simulink model "Utkarsh_2005574_R_W1_P1"  (R2021a)
settings: Solver=VariableStepAuto  StartTime=0.0  StopTime=10.0  RelTol=1e-3
PostLoadFcn:
  | M1=100;
  | K1=50;
  | b=50;
  | M2=40;
  | K12=10;
settings Model: Creator=Utkarsh Anand  LastModifiedBy=Utkarsh Anand

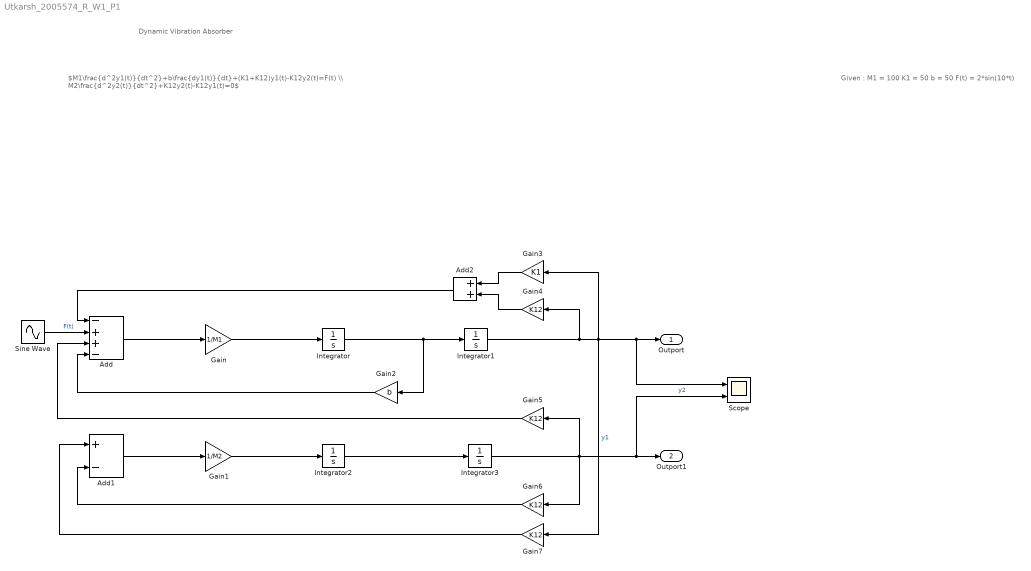
== system Utkarsh_2005574_R_W1_P1 ==
  note: Given :
      | M1 = 100
      | K1 = 50
      | b = 50
      | F(t) = 2*sin(10*t)
  note: $M1\frac{d^2y1(t)}{dt^2}+b\frac{dy1(t)}{dt}+(K1+K12)y1(t)-K12y2(t)=F(t) \\ M2\frac{d^2y2(t)}{dt^2}+K12y2(t)-K12y1(t)=0$
  note: Dynamic Vibration Absorber
  Add : Sum  Inputs=-++-
  Add1 : Sum  Inputs=+-
  Add2 : Sum
  Gain : Gain  Gain=1/M1
  Gain1 : Gain  Gain=1/M2
  Gain2 : Gain  Gain=b
  Gain3 : Gain  Gain=K1
  Gain{4..7} (4 alike) : Gain  Gain=K12
  Integrator{,1..3} (4 alike) : Integrator
  Scope : Scope  NumInputPorts=2
  Sine Wave : Sin  Amplitude=2  Frequency=10  SampleTime=0
  Outport : Outport
  Outport1 : Outport  Port=2
  wires:
  Integrator/1 -> Gain2/1, Integrator1/1
  Gain4/1 -> Add2/2
  Gain3/1 -> Add2/1
  Integrator2/1 -> Integrator3/1
  Integrator3/1 -> Gain6/1, Gain5/1, Scope/2, Outport1/1  "y2"
  Gain6/1 -> Add1/2
  Gain/1 -> Integrator/1
  Add/1 -> Gain/1
  Gain1/1 -> Integrator2/1
  Integrator1/1 -> Gain7/1, Gain3/1, Scope/1, Outport/1, Gain4/1  "y1"
  Gain2/1 -> Add/4
  Add1/1 -> Gain1/1
  Gain7/1 -> Add1/1
  Gain5/1 -> Add/3
  Add2/1 -> Add/1
  Sine Wave/1 -> Add/2  "F(t)"
